simulink model "sim_projekt4_scenariusz1_1"  (R2023b)
settings: Solver=VariableStepAuto  StartTime=0.0  StopTime=10.0  MaxStep=0.01  RelTol=1e-3
undefined symbols (not defined in the file): delta_Twew_SP, k, ki, kp, T, T_wew0, t_wew_SP, T_wew_SP_0, To
settings Model: Creator=tomasz  LastModifiedBy=tomasz

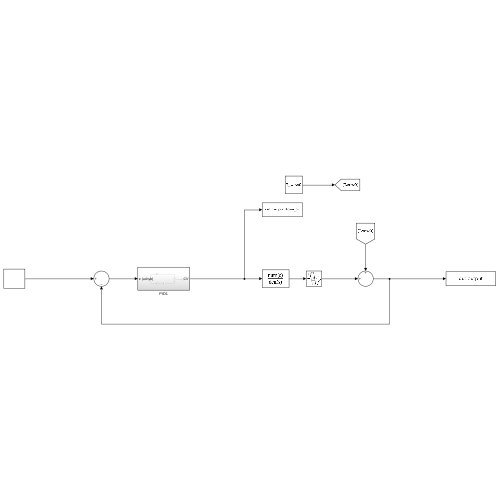
[thumbnail: Simulink's stored preview of the top-level diagram]
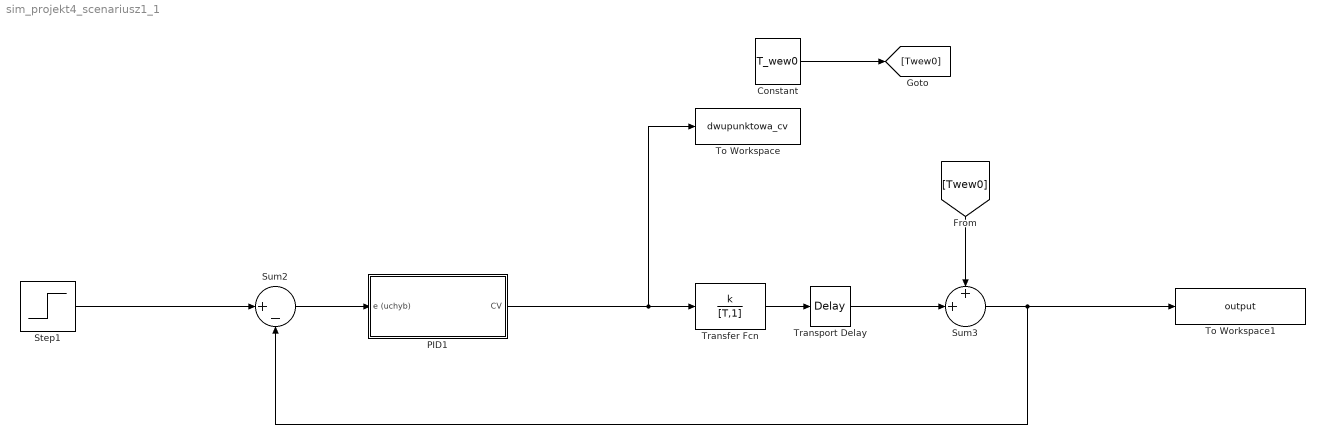
== system sim_projekt4_scenariusz1_1 ==
  Constant : Constant  Value=T_wew0
  PID1 : Subsystem
  Step1 : Step  Time=t_wew_SP  Before=T_wew_SP_0  After=T_wew_SP_0 + delta_Twew_SP  SampleTime=0
  Sum2 : Sum  Inputs=|+-
  Sum3 : Sum  Inputs=++|
  To Workspace : ToWorkspace  VariableName=dwupunktowa_cv  SampleTime=-1
  To Workspace1 : ToWorkspace  VariableName=output  SampleTime=-1
  Transfer Fcn : TransferFcn  Numerator=k  Denominator=[T,1]
  Transport Delay : TransportDelay  DelayTime=To
  wires:
  Sum2/1 -> PID1/1(e (uchyb))
  Sum3/1 -> Sum2/2, To Workspace1/1
  Constant/1 -> [Twew0]
  Transfer Fcn/1 -> Transport Delay/1
  Transport Delay/1 -> Sum3/2
  PID1/1(CV) -> To Workspace/1, Transfer Fcn/1
  Step1/1 -> Sum2/1
  [Twew0] -> Sum3/1

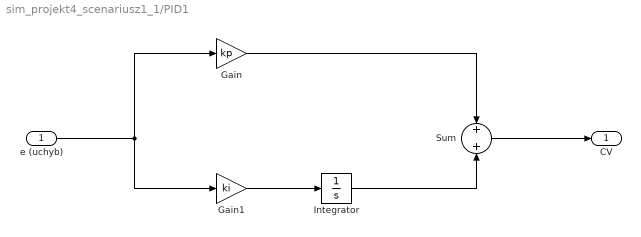
== system sim_projekt4_scenariusz1_1/PID1 ==
  e (uchyb) : Inport
  Gain : Gain  Gain=kp
  Gain1 : Gain  Gain=ki
  Integrator : Integrator
  Sum : Sum
  CV : Outport
  wires:
  Integrator/1 -> Sum/2
  Gain1/1 -> Integrator/1
  Gain/1 -> Sum/1
  e (uchyb)/1 -> Gain1/1, Gain/1
  Sum/1 -> CV/1
